simulink model "chap3_7sim"  (Simulink 6.3)
settings: Solver=ode45  StartTime=0.0  StopTime=2000  RelTol=1e-3
undefined symbols (not defined in the file or in its folder): denP, numP
libraries: simulink x3, powerlib_extras x1
settings Model: Creator=hp  LastModifiedBy=Administrator  ExtModeTrigMode=oneshot  ExtModeArmWhenConnect=off
settings DataIOCC: LimitDataPoints=off
settings OptimizationCC: BlockReduction=off  BooleanDataType=off
settings DebuggingCC: SolverPrmCheckMsg=none
settings HardwareCC: TargetUnknown=on

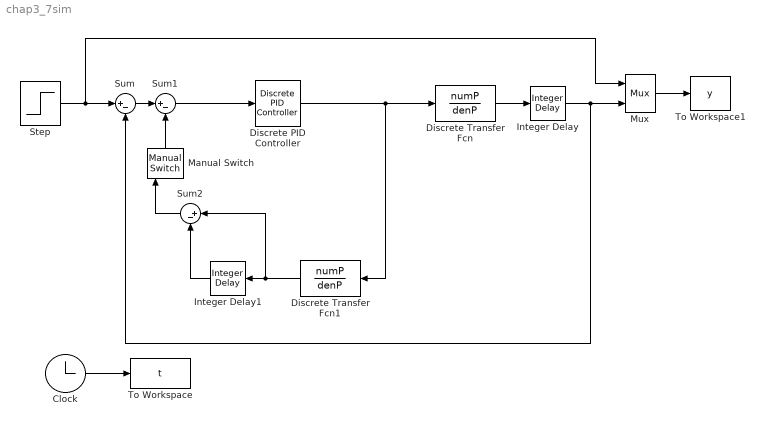
== system chap3_7sim ==
  Clock : Clock
      settings: Decimation=10
  Discrete PID Controller : powerlib_extras/Discrete  Control Blocks/Discrete PID Controller  Kp=0.5  Ki=0.01  Kd=0  TcD=0  Par_Limits=[1e6 -1e6]  Init=0  Ts=20
  Discrete Transfer Fcn : DiscreteTransferFcn  Numerator=numP  Denominator=denP  SampleTime=20
  Discrete Transfer Fcn1 : DiscreteTransferFcn  Orientation=left  Numerator=numP  Denominator=denP  SampleTime=20
  Integer Delay : simulink/Discrete/Integer Delay  vinit=0.0  samptime=20  NumDelays=4
  Integer Delay1 : simulink/Discrete/Integer Delay  Orientation=left  vinit=0.0  samptime=20  NumDelays=4
  Manual Switch : simulink/Signal Routing/Manual Switch  Orientation=up  sw=0  action=0
  Mux : Mux  Inputs=2
  Step : Step  Time=0  SampleTime=20
  Sum : Sum  Inputs=|+-  SaturateOnIntegerOverflow=on  InputSameDT=on
  Sum1 : Sum  Inputs=|+-  SaturateOnIntegerOverflow=on  InputSameDT=on
  Sum2 : Sum  Orientation=left  Inputs=|+-  SaturateOnIntegerOverflow=on  InputSameDT=on
  To Workspace : ToWorkspace  VariableName=t  SampleTime=-1  SaveFormat=Array
  To Workspace1 : ToWorkspace  VariableName=y  SampleTime=20  SaveFormat=Array
  wires:
  Discrete PID Controller/1 -> Discrete Transfer Fcn/1, Discrete Transfer Fcn1/1
  Discrete Transfer Fcn1/1 -> Sum2/1, Integer Delay1/1
  Sum/1 -> Sum1/1
  Step/1 -> Sum/1, Mux/1
  Sum1/1 -> Discrete PID Controller/1
  Integer Delay1/1 -> Sum2/2
  Discrete Transfer Fcn/1 -> Integer Delay/1
  Integer Delay/1 -> Mux/2, Sum/2
  Mux/1 -> To Workspace1/1
  Clock/1 -> To Workspace/1
  Sum2/1 -> Manual Switch/1
  Manual Switch/1 -> Sum1/2
